simulink model "PIDModel_CIMMotor_ConstantRate"  (R2019b)
settings: Solver=VariableStepAuto  StartTime=0.0  StopTime=0.1  RelTol=1e-3
libraries: fl_lib x6, nesl_utility x5, ee_lib x1, simulink x1
settings Model: Creator=chmor  LastModifiedBy=chmor

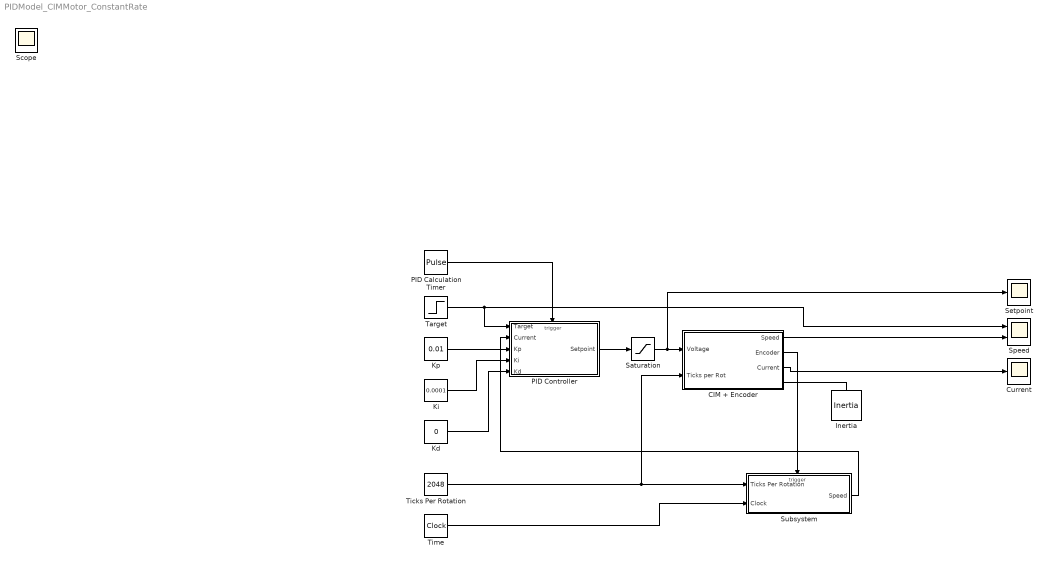
== system PIDModel_CIMMotor_ConstantRate ==
  CIM + Encoder : Subsystem
  Current : Scope
  Inertia : fl_lib/Mechanical/Rotational Elements/Inertia  inertia=0.5*500*5^2 g*cm^2  w_specify=off  w_priority=High  w=0 rad/s  w_nominal_specify=off  w_nominal_unit=rad/s  w_nominal_value=1  t_specify=off  t_priority=None  t=0 N*m  t_nominal_specify=off  t_nominal_unit=N*m  t_nominal_value=1
  Kd : Constant  Value=0
  Ki : Constant  Value=0.0001
  Kp : Constant  Value=0.01
  PID Calculation Timer : DiscretePulseGenerator  PulseType=Time based  Period=0.001  PulseWidth=50
  PID Controller : Subsystem
  Saturation : Saturate  UpperLimit=12  LowerLimit=-12
  Setpoint : Scope
  Speed : Scope  NumInputPorts=2
  Subsystem : Subsystem
  Target : Step  Time=0  After=1000  SampleTime=0
  Ticks Per Rotation : Constant  Value=2048
  Time : DigitalClock  SampleTime=1e-7
  Scope : Scope
  wires:
  Target/1 -> Speed/1, PID Controller/1(Target)
  CIM + Encoder/1(Speed) -> Speed/2
  Kp/1 -> PID Controller/3(Kp)
  Ki/1 -> PID Controller/4(Ki)
  Kd/1 -> PID Controller/5(Kd)
  PID Controller/1(Setpoint) -> Saturation/1
  Ticks Per Rotation/1 -> CIM + Encoder/2(Ticks per Rot), Subsystem/1(Ticks Per Rotation)
  Saturation/1 -> Setpoint/1, CIM + Encoder/1(Voltage)
  CIM + Encoder/3(Current) -> Current/1
  Time/1 -> Subsystem/2(Clock)
  CIM + Encoder/2(Encoder) -> Subsystem/Trigger
  Subsystem/1(Speed) -> PID Controller/2(Current)
  PID Calculation Timer/1 -> PID Controller/Trigger
  connections:
  CIM + Encoder/RConn1 -- Inertia/LConn1

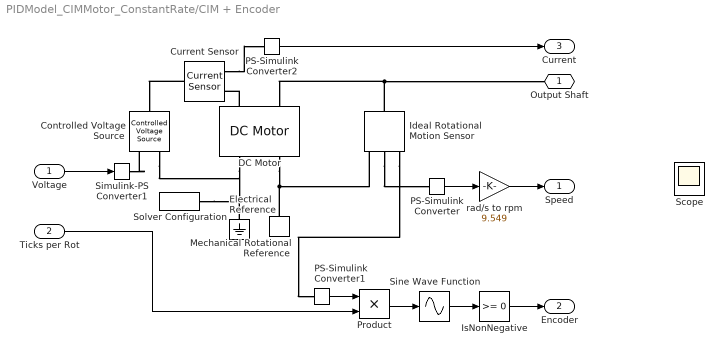
== system PIDModel_CIMMotor_ConstantRate/CIM + Encoder ==
  Voltage : Inport
  Ticks per Rot : Inport  Port=2
  Controlled Voltage Source : fl_lib/Electrical/Electrical Sources/Controlled Voltage Source
  Current Sensor : fl_lib/Electrical/Electrical Sensors/Current Sensor
  DC Motor : ee_lib/Electromechanical/Brushed Motors/DC Motor  parameterization=2  Ra=0.0916 Ohm  La=59 uH  emf_or_torque=2  Kv=0.072e-3 V/rpm  Ki=0.0184 N*m/A  T_stall=2.4249 N*m  w_max=5330 rpm  w_rated=15000 rpm  P_rated=0.08 W  V_rated=12 V  J=7.75e-5 kg*m^2  lam_param=2  lam=0 N*m/(rad/s)  i_noload=2.7 A  V_i_noload=12 V  speed0=0 rpm  alpha=3.93e-3 1/K  Tmeas=25 degC  thermal_mass=100 J/K  initial_temperature=25 degC
      settings: SourceProductName=Simscape Electrical
  Electrical Reference : fl_lib/Electrical/Electrical Elements/Electrical Reference
  Ideal Rotational Motion Sensor : fl_lib/Mechanical/Mechanical Sensors/Ideal Rotational Motion Sensor  offset=0 deg
  IsNonNegative : simulink/Logic and Bit Operations/Compare To Zero  relop=>=  OutDataTypeStr=boolean
  Mechanical Rotational Reference : fl_lib/Mechanical/Rotational Elements/Mechanical Rotational Reference
  PS-Simulink Converter : nesl_utility/PS-Simulink Converter  PhysicalDomain=network_engine_domain  SubClassName=ps_output  LeftPortType=input  RightPortType=output  PseudoPeriodic=off  Frequencies=[]  Unit=inherit  AffineConversion=off
  PS-Simulink Converter1 : nesl_utility/PS-Simulink Converter  PhysicalDomain=network_engine_domain  SubClassName=ps_output  LeftPortType=input  RightPortType=output  PseudoPeriodic=off  Frequencies=[]  Unit=inherit  AffineConversion=off
  PS-Simulink Converter2 : nesl_utility/PS-Simulink Converter  PhysicalDomain=network_engine_domain  SubClassName=ps_output  LeftPortType=input  RightPortType=output  PseudoPeriodic=off  Frequencies=[]  Unit=inherit  AffineConversion=off
  Product : Product
  Scope : Scope  NumInputPorts=2
  Simulink-PS Converter1 : nesl_utility/Simulink-PS Converter  PhysicalDomain=network_engine_domain  SubClassName=ps_input  LeftPortType=input  RightPortType=output  PseudoPeriodic=off  Frequencies=[]  NoiseDistribution=none  NoiseParameters=[]  Unit=1  AffineConversion=off  FilteringAndDerivatives=provide  SimscapeFilterOrder=1  InputFilterTimeConstant=0.001  UdotUserProvided=0
  Sine Wave Function : Sin  TimeSource=Use external signal  SampleTime=0
  Solver Configuration : nesl_utility/Solver Configuration  PhysicalDomain=network_engine_domain  SubClassName=solver  LeftPortType=input  RightPortType=generic  Tones=[]  Harmonics=[]  SimulateNoise=off  Profile=off  UseLocalSampling=off  EnableSwitchedLinearOptims=on  FrequencyDomain=off  UseCCode=off  RelTol=0.001  AbsTol=1e-06  MinStep=1e-09  ToWorkspace=off  RevertToSquareIcSolve=off  NumHomotopyIterations=100  PhasorMode=off  PhasorModeNumHarmonics=1  DoDC=off  ResidualTolerance=1e-09  UseLocalSolver=off  LocalSolverChoice=NE_BACKWARD_EULER_ADVANCER  LocalSolverSampleTime=0.001  DoFixedCost=off  MaxNonlinIter=3  MaxModeIter=2  LinearAlgebra=auto  EquationFormulation=NE_TIME_EF  DelaysMemoryBudget=1024  AutomaticFiltering=on  FilteringTimeConstant=0.001  PartitionStorageMethod=AS_NEEDED  PartitionMemoryBudget=1024  PartitionMethod=ROBUST
  rad/s to rpm : Gain  Gain=9.549
  Output Shaft : PMIOPort  Side=Right
  Speed : Outport
  Encoder : Outport  Port=2
  Current : Outport  Port=3
  wires:
  Voltage/1 -> Simulink-PS Converter1/1
  PS-Simulink Converter/1 -> rad/s to rpm/1
  rad/s to rpm/1 -> Speed/1
  Sine Wave Function/1 -> IsNonNegative/1
  Product/1 -> Sine Wave Function/1
  PS-Simulink Converter1/1 -> Product/1
  Ticks per Rot/1 -> Product/2
  IsNonNegative/1 -> Encoder/1
  PS-Simulink Converter2/1 -> Current/1
  connections:
  Simulink-PS Converter1/RConn1 -- Controlled Voltage Source/RConn1
  Ideal Rotational Motion Sensor/RConn2 -- PS-Simulink Converter/LConn1
  Solver Configuration/RConn1 -- Electrical Reference/LConn1 -- Controlled Voltage Source/RConn2 -- DC Motor/RConn1
  DC Motor/RConn2 -- Ideal Rotational Motion Sensor/RConn1 -- Mechanical Rotational Reference/LConn1
  Ideal Rotational Motion Sensor/LConn1 -- Output Shaft/RConn1 -- DC Motor/LConn2
  Ideal Rotational Motion Sensor/RConn3 -- PS-Simulink Converter1/LConn1
  Current Sensor/LConn1 -- Controlled Voltage Source/LConn1
  DC Motor/LConn1 -- Current Sensor/RConn2
  Current Sensor/RConn1 -- PS-Simulink Converter2/LConn1

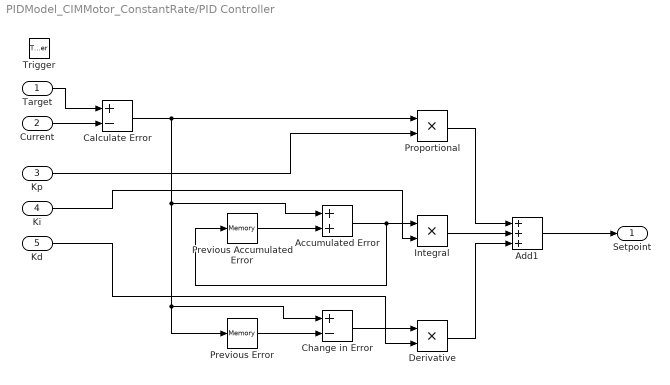
== system PIDModel_CIMMotor_ConstantRate/PID Controller ==
  Target : Inport
  Current : Inport  Port=2
  Kp : Inport  Port=3
  Ki : Inport  Port=4
  Kd : Inport  Port=5
  Trigger : TriggerPort  VariantControl=Variant  SampleTimeType=periodic  SampleTime=0.001  InitialTriggerSignalState=zero  PortDimensions=1
  Accumulated Error : Sum
  Add1 : Sum  Inputs=+++
  Calculate Error : Sum  Inputs=+-
  Change in Error : Sum  Inputs=+-
  Derivative : Product
  Integral : Product
  Previous Accumulated Error : Memory  InheritSampleTime=on
  Previous Error : Memory  InheritSampleTime=on
  Proportional : Product
  Setpoint : Outport  InitialOutput=0
  wires:
  Integral/1 -> Add1/2
  Calculate Error/1 -> Previous Error/1, Change in Error/1, Accumulated Error/1, Proportional/1
  Accumulated Error/1 -> Integral/1, Previous Accumulated Error/1
  Previous Error/1 -> Change in Error/2
  Change in Error/1 -> Derivative/1
  Previous Accumulated Error/1 -> Accumulated Error/2
  Proportional/1 -> Add1/1
  Target/1 -> Calculate Error/1
  Derivative/1 -> Add1/3
  Ki/1 -> Integral/2
  Kp/1 -> Proportional/2
  Kd/1 -> Derivative/2
  Current/1 -> Calculate Error/2
  Add1/1 -> Setpoint/1

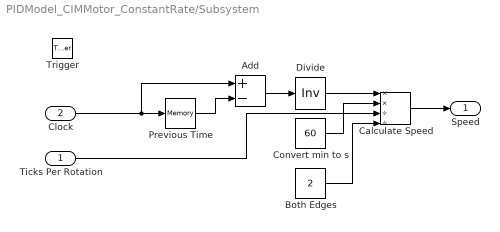
== system PIDModel_CIMMotor_ConstantRate/Subsystem ==
  Ticks Per Rotation : Inport
  Clock : Inport  Port=2
  Trigger : TriggerPort  TriggerType=either  VariantControl=Variant  InitialTriggerSignalState=zero  PortDimensions=1
  Add : Sum  Inputs=+-
  Both Edges : Constant  Value=2
  Calculate Speed : Product  Inputs=**//
  Convert min to s : Constant  Value=60
  Divide : Product  Inputs=/  Multiplication=Matrix(*)
  Previous Time : Memory  InitialCondition=-1  InheritSampleTime=on
  Speed : Outport  InitialOutput=0
  wires:
  Clock/1 -> Add/1, Previous Time/1
  Calculate Speed/1 -> Speed/1
  Add/1 -> Divide/1
  Convert min to s/1 -> Calculate Speed/2
  Previous Time/1 -> Add/2
  Ticks Per Rotation/1 -> Calculate Speed/3
  Divide/1 -> Calculate Speed/1
  Both Edges/1 -> Calculate Speed/4
